simulink model "AscTecTest"  (Simulink 7.6)
settings: Solver=ode3  StartTime=0.0  StopTime=inf  FixedStep=0.05  RelTol=1e-3
libraries: aerolibanimutils x1
settings Model: Creator=Owen  LastModifiedBy=Owen

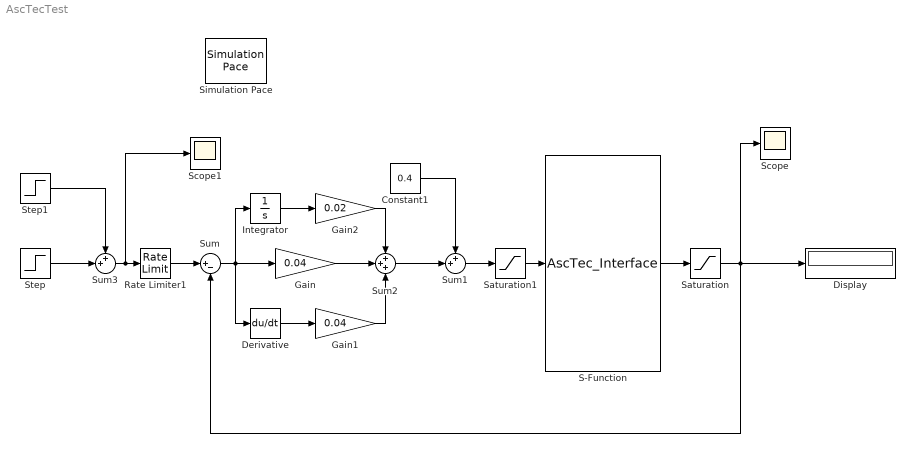
== system AscTecTest ==
  Constant1 : Constant  Value=0.4
  Derivative : Derivative
  Display : Display
  Gain : Gain  Gain=0.04
  Gain1 : Gain  Gain=0.04
  Gain2 : Gain  Gain=0.02
  Integrator : Integrator
  Rate Limiter1 : RateLimiter  RisingSlewLimit=0.1  FallingSlewLimit=-0.1  SampleTimeMode=inherited
  S-Function : S-Function  FunctionName=AscTec_Interface  Parameters='COM5',57600  EnableBusSupport=off
  Saturation : Saturate  UpperLimit=1  LowerLimit=0
  Saturation1 : Saturate  UpperLimit=1  LowerLimit=0
  Scope : Scope
      settings: SaveName=UltraNoise  DataFormat=Array
  Scope1 : Scope
      settings: SaveName=UltraNoise1  DataFormat=Array
  Simulation Pace : aerolibanimutils/Simulation Pace  SimulationPace=1  SleepMode=MATLAB Thread  OutputPaceError=off  SampleTime=0.05
      settings: AttributesFormatString=%<SimulationPace> sec/sec
  Step : Step  Time=5  After=0.4  SampleTime=0
  Step1 : Step  Time=30  After=-0.4  SampleTime=0
  Sum : Sum  Inputs=|+-
  Sum1 : Sum  Inputs=++|
  Sum2 : Sum  Inputs=+++
  Sum3 : Sum  Inputs=++|
  wires:
  S-Function/1 -> Saturation/1
  Sum/1 -> Gain/1, Derivative/1, Integrator/1
  Gain/1 -> Sum2/2
  Constant1/1 -> Sum1/1
  Sum1/1 -> Saturation1/1
  Sum2/1 -> Sum1/2
  Saturation/1 -> Scope/1, Display/1, Sum/2
  Saturation1/1 -> S-Function/1
  Gain1/1 -> Sum2/3
  Derivative/1 -> Gain1/1
  Gain2/1 -> Sum2/1
  Integrator/1 -> Gain2/1
  Step/1 -> Sum3/2
  Sum3/1 -> Scope1/1, Rate Limiter1/1
  Step1/1 -> Sum3/1
  Rate Limiter1/1 -> Sum/1
